simulink library "HX_EN12977_stratified"  (R2018b)
settings: Solver=ode45  StartTime=0.0  StopTime=10.0  RelTol=1e-3  EnableMultiTasking=on
undefined symbols (not defined in the file): height
libraries: carnot x2
settings Model: Creator=lena.frank  LastModifiedBy=drhf
settings DataIOCC: LimitDataPoints=on  SaveFormat=Array  SignalLoggingSaveFormat=ModelDataLogs
settings OptimizationCC: ExpressionDepthLimit=2147483647  LifeSpan=inf
settings DebuggingCC: UnderspecifiedInitializationDetection=Classic  MergeDetectMultiDrivingBlocksExec=none  SolverPrmCheckMsg=warning  FcnCallInpInsideContextMsg=warning  StateNameClashWarn=warning  SFUnexpectedBacktrackingDiag=warning  SFNoUnconditionalDefaultTransitionDiag=warning  SFExecutionAtInitializationDiag=none
settings HardwareCC: ProdBitPerPointer=32  ProdBitPerSizeT=32  ProdBitPerPtrDiffT=32  ProdLargestAtomicFloat=None  ProdIntDivRoundTo=Undefined  ProdEndianess=Unspecified  ProdWordSize=32  ProdHWDeviceType=32-bit Generic
settings ModelReferenceCC: PropagateSignalLabelsOutOfModel=off
settings SFSimCC: SimUseLocalCustomCode=off
settings RTWCC: RTWUseLocalCustomCode=off
settings CodeAppCC: StateflowObjectComments=on
settings GRTTargetCC: TargetLangStandard=C89/C90 (ANSI)  GeneratePreprocessorConditionals=Disable all  CombineOutputUpdateFcns=off  GRTInterface=on
settings ConfigComp: CovMetricSettings=dw  CovHtmlReporting=on  CovSaveCumulativeToWorkspaceVar=on  CovSaveSingleToWorkspaceVar=on  CovExternalEMLEnable=off

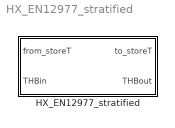
== system HX_EN12977_stratified ==
  HX_EN12977_stratified : Subsystem  mask(stratified heat exchanger for storage, data EN 12977){h_in=1, h_out=0, hgt=height, dia=0.03, height=, ua0=100, uam=0.1, uat=0.5, uat2=0, dplin=100, dpqua=100, nodes=10}
      mask prompts: h_in "relative height of inlet"; h_out "relative height of outlet"; hgt "Height of storage in m"; dia "Diameter of HX pipe [m]"; height "Height difference inlet-outlet [m]"; ua0 "uac: heat transfer coefficient [W/K /(kg/s) /(°C)]"; uam "uam: massflow dependent heat transfer [-]"; uat "uat: temperature dependent heat transfer [-]"; uat2 "uat2: temperature difference dependent heat transfer [-]"; dplin "Pressure drop coefficient dplin [Pa/(kg/s)]"; dpqua "Pressure drop coefficient dpqua [Pa/(kg/s)²]"; nodes "number of nodes"
      mask help:
      | The block transforms the incoming THV vector to a vector which the storage interprets as a heat exchanger.
      | Give inlet and outlet as a relative position 0=bottom to 1=top
      | The heat transfer is calculated by:
      | UA = uac * mdot^uam *
      |           ((Theatexchanger+Tstorage)/2)^uat *
      |           (Theatexchanger-Tstorage)^uat2
      | Stratified:
      | For charging (inlet above outlet) the heat transfer starts when the storage temperature is below the heat exchanger temperature.
      | For discharging (outlet above inlet) the heat transfer starts when the storage temperature is above the heat exchanger temperature.
      mask init:
      | in = zeros(nodes,1);    % vector of length nodes
      | up = in;                % vector of length nodes
      | down = in;              % vector of length nodes
      | 
      | h_in = max(0,h_in);     % no nodes below 0
      | h_out = max(0,h_out);   % no nodes below 0
      | 
      | inlet = round(h_in*(nodes-1))+1;    % inlet position
      | outlet = round(h_out*(nodes-1))+1;  % outlet position
      | set_param(gcb,'height',num2str((h_out-h_in)*hgt));
      | % hgt = (h_out-h_in)*hgt;
      | 
      | in(inlet)=1;
      | 
      | if (h_in < h_out)           % if inlet below outlet
      |     up(inlet:outlet)=1;     % upwards
      | elseif (h_in > h_out)       % else if inlet above outlet
      |     down(outlet:inlet)=1;   % downwards
      | end
      mask Help: web(['file:///' fullfile(path_carnot('help'),'StoragePorts_HeatExchangerModels.html')],'-helpbrowser')
      mask TypeOptions dia: Pressure_Drop_StorageHX/dia
      mask TypeOptions height: Pressure_Drop_StorageHX/hgt
      mask TypeOptions ua0: sfun_storage_heatexchanger/p1
      mask TypeOptions uam: sfun_storage_heatexchanger/p2
      mask TypeOptions uat: sfun_storage_heatexchanger/p3
      mask TypeOptions uat2: sfun_storage_heatexchanger/p4
      mask TypeOptions dplin: Pressure_Drop_StorageHX/dplin
      mask TypeOptions dpqua: Pressure_Drop_StorageHX/dpqua
      mask TypeOptions nodes: sfun_storage_heatexchanger/nodes
      mask DialogControl ParameterTabVar0 Prompt: Geometry
      mask DialogControl ParameterTabVar01 Prompt: Heat transfer
      mask DialogControl ParameterTabVar012 Prompt: Pressure drop
      mask DialogControl ParameterTabVar0123 Prompt: Calculation
      mask Display: disp('HX EN12977 STRAT')

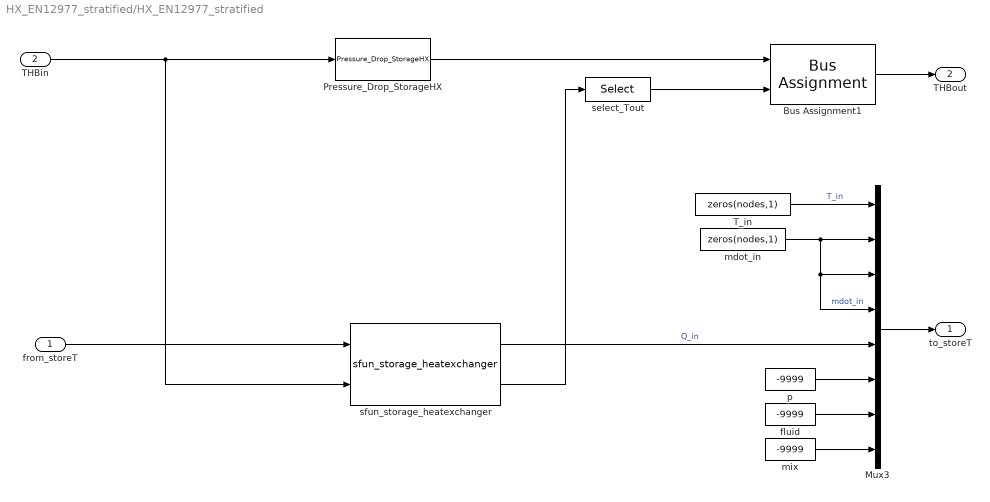
== system HX_EN12977_stratified/HX_EN12977_stratified ==
  from_storeT : Inport
  THBin : Inport  Port=2
  Bus Assignment1 : BusAssignment  AssignedSignals=Temperature
  Mux3 : Mux  Inputs=8
  Pressure_Drop_StorageHX : carnot/Basic/Pressure_Drop/Pressure_Drop_StorageHX  dia=dia  hgt=height  dplin=dplin  dpqua=dpqua
      settings: SourceProductName=Carnot
  T_in : Constant  Value=zeros(nodes,1)
  fluid : Constant  Value=-9999
  mdot_in : Constant  Value=zeros(nodes,1)
  mix : Constant  Value=-9999
  p : Constant  Value=-9999
  select_Tout : Selector  InputPortWidth=nodes  IndexOptions=Index vector (dialog)  Indices=[outlet]  OutputSizes=1
  sfun_storage_heatexchanger : carnot/Basic/Thermal_Models/sfun_storage_heatexchanger  idn="heat transfer data fit EN12977  - stratified"  nodes=nodes  inlet=inlet  outlet=outlet  p1=ua0  p2=uam  p3=uat  p4=uat2  p5=0  p6=0  p7=0
      settings: SourceProductName=Carnot
  to_storeT : Outport
  THBout : Outport  Port=2
  wires:
  Pressure_Drop_StorageHX/1 -> Bus Assignment1/1
  sfun_storage_heatexchanger/2 -> select_Tout/1
  mix/1 -> Mux3/8
  fluid/1 -> Mux3/7
  p/1 -> Mux3/6
  Bus Assignment1/1 -> THBout/1
  sfun_storage_heatexchanger/1 -> Mux3/5  "Q_in"
  T_in/1 -> Mux3/1  "T_in"
  select_Tout/1 -> Bus Assignment1/2
  Mux3/1 -> to_storeT/1
  mdot_in/1 -> Mux3/4, Mux3/3, Mux3/2  "mdot_in"
  THBin/1 -> sfun_storage_heatexchanger/2, Pressure_Drop_StorageHX/1
  from_storeT/1 -> sfun_storage_heatexchanger/1
